simulink model "controlAerobi"  (R2017b)
settings: Solver=FixedStepDiscrete  StartTime=0.0  StopTime=inf  FixedStep=Ts  RelTol=1e-3
InitFcn:
  | load Navio2_bus;
  | Ts=0.0025;
StopFcn:
  | %save_system('controlAerobi.slx');
  | %run('D:\Eclipse_Workspaces\workspace_rasp\AutoPilot\contAerobi\UpdateFiles\CopyBuildFiles.m');
undefined symbols (not defined in the file or in its folder): DiscIntNeverNeededParam
libraries: simulink x36, sharedutil x1, sharedtransform x1, dspsigops x1
(part 3 of 4)

== system controlAerobi/Controllers/Quadrotor_Controllers/PID_cascade_controllers/PID_ATTITUDE_CONTROLLER/PID_yaw/Clamping circuit1 ==
  preSat : Inport
  postSat : Inport  Port=2
  preIntegrator : Inport  Port=3
  AND : Logic  DisableCoverage=on  OutDataTypeStr=boolean
  Abs : Abs
  Add : Sum  Inputs=+-
  Compare To Constant : simulink/Logic and Bit Operations/Compare To Constant  relop=>=  const=1e-10  OutDataTypeStr=boolean
  Equal : RelationalOperator  DisableCoverage=on  Operator===  OutDataTypeStr=boolean  RndMeth=Nearest  InputSameDT=on
  SignPreIntegrator : Signum  DisableCoverage=on
  SignPreSat : Signum  DisableCoverage=on
  Clamp : Outport
  wires:
  Abs/1 -> Compare To Constant/1
  Add/1 -> Abs/1
  postSat/1 -> Add/2
  preSat/1 -> Add/1, SignPreSat/1
  preIntegrator/1 -> SignPreIntegrator/1
  SignPreSat/1 -> Equal/1
  Compare To Constant/1 -> AND/1
  SignPreIntegrator/1 -> Equal/2
  Equal/1 -> AND/2
  AND/1 -> Clamp/1

== system controlAerobi/Controllers/Quadrotor_Controllers/PID_cascade_controllers/PID_POSITION_CONTROLLER/XY_controller/PID_XY ==
  Error : Inport
  Reset : Inport  Port=2
  ControlParam : Inport  Port=3
  Bus Selector : BusSelector  OutputSignals=PIDgains.XYcontroller.P_pos,PIDgains.XYcontroller.I_pos,PIDgains.XYcontroller.D_pos,PIDgains.XYcontroller.Sat+_XY_pos,PIDgains.XYcontroller.Sat-_XY_pos
  Clamping circuit1 : Subsystem
  Constant : Constant  Value=0
  Constant1 : Constant  Value=0
  Discrete Derivative : simulink/Discrete/Discrete Derivative  gainval=1.0  ICPrevScaledInput=0.0  InputProcessing=Inherited  OutMin=[]  OutMax=[]  OutDataType=fixdt(1, 16)  OutScaling=2^-10  DoSatur=off
  Discrete-Time Integrator : DiscreteIntegrator  ExternalReset=rising  SampleTime=Ts  ICPrevOutput=DiscIntNeverNeededParam  ICPrevScaledInput=DiscIntNeverNeededParam
  Product : Product  RndMeth=Zero
  Product1 : Product  RndMeth=Zero
  Product2 : Product  RndMeth=Zero
  Saturation Dynamic : simulink/Discontinuities/Saturation Dynamic  OutMin=[]  OutMax=[]  OutDataTypeStr=Inherit: Same as second input  OutDataType=fixdt(1, 16)  OutScaling=2^-10  DoSatur=off
  Sum : Sum  Inputs=+++
  Switch : Switch  Criteria=u2 > Threshold
  Switch4 : Switch  Criteria=u2 ~= 0
  dxdy_des : Outport
  wires:
  Error/1 -> Switch4/1
  Switch4/1 -> Product2/2, Product/2, Product1/2
  Constant1/1 -> Switch4/3
  Bus Selector/5 -> Saturation Dynamic/3  "<Sat-_XY_pos>"
  Bus Selector/4 -> Saturation Dynamic/1  "<Sat+_XY_pos>"
  Bus Selector/3 -> Product2/1  "<D_pos>"
  Bus Selector/2 -> Product1/1  "<I_pos>"
  Bus Selector/1 -> Product/1  "<P_pos>"
  ControlParam/1 -> Bus Selector/1
  Discrete Derivative/1 -> Sum/3
  Product2/1 -> Discrete Derivative/1
  Product/1 -> Sum/1
  Sum/1 -> Saturation Dynamic/2, Clamping circuit1/1(preSat)
  Reset/1 -> Switch4/2, Discrete-Time Integrator/2
  Discrete-Time Integrator/1 -> Sum/2
  Saturation Dynamic/1 -> dxdy_des/1, Clamping circuit1/2(postSat)
  Switch/1 -> Discrete-Time Integrator/1
  Clamping circuit1/1(Clamp) -> Switch/2
  Product1/1 -> Switch/3, Clamping circuit1/3(preIntegrator)
  Constant/1 -> Switch/1

== system controlAerobi/Controllers/Quadrotor_Controllers/PID_cascade_controllers/PID_POSITION_CONTROLLER/XY_controller/PID_dXY ==
  Error : Inport
  Reset : Inport  Port=2
  ControlGains : Inport  Port=3
  Bus Selector : BusSelector  OutputSignals=PIDgains.XYcontroller.P_rate,PIDgains.XYcontroller.I_rate,PIDgains.XYcontroller.D_rate,PIDgains.XYcontroller.Sat+_rate,PIDgains.XYcontroller.Sat-_rate
  Clamping circuit1 : Subsystem
  Constant : Constant  Value=0
  Constant1 : Constant  Value=0
  Discrete Derivative : simulink/Discrete/Discrete Derivative  gainval=1.0  ICPrevScaledInput=0.0  InputProcessing=Inherited  OutMin=[]  OutMax=[]  OutDataType=fixdt(1, 16)  OutScaling=2^-10  DoSatur=off
  Discrete-Time Integrator : DiscreteIntegrator  ExternalReset=rising  SampleTime=Ts  ICPrevOutput=DiscIntNeverNeededParam  ICPrevScaledInput=DiscIntNeverNeededParam
  Product : Product  RndMeth=Zero
  Product1 : Product  RndMeth=Zero
  Product2 : Product  RndMeth=Zero
  Saturation Dynamic : simulink/Discontinuities/Saturation Dynamic  OutMin=[]  OutMax=[]  OutDataTypeStr=Inherit: Same as second input  OutDataType=fixdt(1, 16)  OutScaling=2^-10  DoSatur=off
  Sum : Sum  Inputs=+++
  Switch : Switch  Criteria=u2 > Threshold
  Switch4 : Switch  Criteria=u2 ~= 0
  Fx/Fy : Outport
  wires:
  Constant/1 -> Switch/1
  Product1/1 -> Clamping circuit1/3(preIntegrator), Switch/3
  Clamping circuit1/1(Clamp) -> Switch/2
  Switch/1 -> Discrete-Time Integrator/1
  Saturation Dynamic/1 -> Clamping circuit1/2(postSat), Fx/Fy/1
  Discrete-Time Integrator/1 -> Sum/2
  Reset/1 -> Discrete-Time Integrator/2, Switch4/2
  Sum/1 -> Clamping circuit1/1(preSat), Saturation Dynamic/2
  Product/1 -> Sum/1
  Product2/1 -> Discrete Derivative/1
  Discrete Derivative/1 -> Sum/3
  ControlGains/1 -> Bus Selector/1
  Bus Selector/1 -> Product/1  "<P_rate>"
  Bus Selector/2 -> Product1/1  "<I_rate>"
  Bus Selector/3 -> Product2/1  "<D_rate>"
  Bus Selector/4 -> Saturation Dynamic/1  "<Sat+_rate>"
  Bus Selector/5 -> Saturation Dynamic/3  "<Sat-_rate>"
  Constant1/1 -> Switch4/3
  Switch4/1 -> Product1/2, Product/2, Product2/2
  Error/1 -> Switch4/1

== system controlAerobi/Controllers/Quadrotor_Controllers/PID_cascade_controllers/PID_POSITION_CONTROLLER/XY_controller/create_references ==
  yaw : Inport
  ControlModes : Inport  Port=2
  Bus Selector1 : BusSelector  OutputSignals=RemoteControl.Pitch/Xdes,RemoteControl.Roll/Ydes,ModeControl.RESET,ModeControl.POS_HOLD,ModeControl.Pos/VelXY
  Create dXY desired : MATLAB Function  TreatAsAtomicUnit=on
  Dead Zone : DeadZone  LowerValue=-0.05  UpperValue=0.05  SaturateOnIntegerOverflow=on
  Dead Zone1 : DeadZone  LowerValue=-0.05  UpperValue=0.05  SaturateOnIntegerOverflow=on
  Gain : Gain  Gain=-3
  Gain1 : Gain  Gain=3
  Logical Operator : Logic  AllPortsSameDT=off  OutDataTypeStr=boolean
  Saturation1 : Saturate  UpperLimit=3  LowerLimit=-3
  Switch1 : Switch  Criteria=u2 ~= 0
  antiwind_up_xydes : Subsystem
  zero : Constant  Value=0
  dXY_ref : Outport
  XY_ref : Outport  Port=2
  signal : Outport  Port=3
  reset : Outport  Port=4
  <POS_HOLD> : Outport  Port=5
  <Pos/VelXY> : Outport  Port=6
  wires:
  ControlModes/1 -> Bus Selector1/1
  Gain/1 -> Create dXY desired/2(chan2)
  Gain1/1 -> Create dXY desired/3(chan3)
  Bus Selector1/3 -> Logical Operator/1  "<RESET>"
  Bus Selector1/4 -> <POS_HOLD>/1, Logical Operator/2  "<POS_HOLD>"
  Bus Selector1/1 -> Dead Zone/1  "<Pitch/Xdes>"
  Bus Selector1/2 -> Dead Zone1/1  "<Roll/Ydes>"
  Bus Selector1/5 -> Switch1/2, <Pos/VelXY>/1  "<Pos/VelXY>"
  Dead Zone/1 -> Gain/1
  Dead Zone1/1 -> Gain1/1
  Logical Operator/1 -> antiwind_up_xydes/2(reset), reset/1
  Create dXY desired/1(dXY_d) -> Saturation1/1
  Saturation1/1 -> dXY_ref/1, Switch1/1
  yaw/1 -> Create dXY desired/1(yaw)
  Switch1/1 -> antiwind_up_xydes/1(error)
  zero/1 -> Switch1/3
  antiwind_up_xydes/1(ref) -> XY_ref/1
  antiwind_up_xydes/2(signal) -> signal/1

== system controlAerobi/Controllers/Quadrotor_Controllers/PID_cascade_controllers/PID_POSITION_CONTROLLER/Z_controller/Altitude_PIDs ==
  TI : Inport
  Zdes : Inport  Port=2
  dZdes : Inport  Port=3
  ControlGains : Inport  Port=4
  DataSensor : Inport  Port=5
  ControlModes : Inport  Port=6
  Bus Creator : BusCreator  Inputs=2
  Bus Selector : BusSelector  OutputSignals=position_.Position.z,position_.Velocity.dz,attitude_.AngularPosition.roll,attitude_.AngularPosition.pitch
  Bus Selector1 : BusSelector  OutputSignals=ModeControl.ALTHOLD,ModeControl.Pos/VelZ
  Divide : Product  Inputs=*/
  PID_Z : Subsystem
  PID_dZ : Subsystem
  Product : Product  RndMeth=Zero
  Sum1 : Sum  Inputs=|+-
  Sum2 : Sum
  Sum5 : Sum  Inputs=|+-
  Switch1 : Switch  Criteria=u2 ~= 0
  Trigonometric Function : Trigonometry  Operator=cos
  Trigonometric Function1 : Trigonometry  Operator=cos
  T : Outport
  dZ_des : Outport  Port=2
  wires:
  Sum5/1 -> PID_dZ/1(Error)
  PID_Z/1(dZ_des) -> Switch1/1
  Switch1/1 -> Sum5/1, Bus Creator/2  "dZ_des"
  Bus Selector/2 -> Sum5/2  "<dz>"
  Sum1/1 -> PID_Z/1(Error)
  PID_dZ/1(Fz) -> Sum2/2
  Zdes/1 -> Sum1/1, Bus Creator/1  "Z_des"
  Bus Selector1/1 -> PID_dZ/2(Reset), PID_Z/2(Reset)  "<ALTHOLD>"
  Sum2/1 -> Divide/1
  Product/1 -> Divide/2
  Trigonometric Function/1 -> Product/1
  Trigonometric Function1/1 -> Product/2
  Divide/1 -> T/1
  TI/1 -> Sum2/1
  Bus Selector/3 -> Trigonometric Function/1  "<roll>"
  Bus Selector/4 -> Trigonometric Function1/1  "<pitch>"
  DataSensor/1 -> Bus Selector/1
  ControlGains/1 -> PID_dZ/3(ControlGains), PID_Z/3(ControlGains)
  Bus Creator/1 -> dZ_des/1
  dZdes/1 -> Switch1/3
  Bus Selector/1 -> Sum1/2  "<z>"
  ControlModes/1 -> Bus Selector1/1
  Bus Selector1/2 -> Switch1/2  "<Pos/VelZ>"

== system controlAerobi/Controllers/Quadrotor_Controllers/PID_cascade_controllers/PID_POSITION_CONTROLLER/Z_controller/calculate_altitude_des ==
  DataSensor : Inport
  ControlModes : Inport  Port=2
  Bus Selector : BusSelector  OutputSignals=PositionDesired.Zdes,ModeControl.Pos/VelZ,ModeControl.EnablePC,RemoteControl.Thrust/Zdes,ModeControl.ALTHOLD
  Bus Selector1 : BusSelector  OutputSignals=position_.Position.z
  Saturation : Saturate  UpperLimit=inf  LowerLimit=0
  Sum : Sum  Inputs=|+-
  Sum1 : Sum  Inputs=|++
  Switch : Switch  Criteria=u2 ~= 0
  altitude_fcn : MATLAB Function  TreatAsAtomicUnit=on
  and : Logic  AllPortsSameDT=off  OutDataTypeStr=boolean
  antiwind_up_dzdes : Subsystem
  antiwind_up_zdes : Subsystem
  med_thrust : Constant  Value=52.23
  T : Outport
  Zdes : Outport  Port=2
  dZdes : Outport  Port=3
  wires:
  ControlModes/1 -> Bus Selector/1
  DataSensor/1 -> Bus Selector1/1
  Bus Selector/2 -> and/1  "<Pos/VelZ>"
  Bus Selector/1 -> Switch/1  "<Zdes>"
  Bus Selector/3 -> and/2  "<EnablePC>"
  and/1 -> Switch/2
  Switch/1 -> Zdes/1
  Bus Selector/5 -> antiwind_up_zdes/2(reset), altitude_fcn/2(althold)  "<ALTHOLD>"
  Bus Selector/4 -> altitude_fcn/3(thrust), Sum/1  "<Thrust/Zdes>"
  med_thrust/1 -> Sum/2
  Bus Selector1/1 -> altitude_fcn/1(z)  "<z>"
  altitude_fcn/1(zdes) -> Sum1/2
  altitude_fcn/2(thrust_ini) -> T/1
  antiwind_up_zdes/1(I) -> Sum1/1
  Sum1/1 -> Saturation/1
  antiwind_up_dzdes/1(I) -> antiwind_up_zdes/1(error), dZdes/1
  Sum/1 -> antiwind_up_dzdes/1(error)
  Saturation/1 -> Switch/3

== system controlAerobi/Controllers/Quadrotor_Controllers/Geometric_controller/trajectory_tracking/Generate_tracking_referecnces/calculate_altitude_des/antiwind_up_dzdes ==
  error : Inport
  1-D Lookup Table : Lookup_n-D  NumberOfTableDimensions=1  BreakpointsForDimension1=[-3:0.01:3]  Table=[-3:0.01:3]  InternalRulePriority=Speed  RndMeth=Simplest  InputSameDT=on
  Dead Zone : DeadZone  LowerValue=-0.8  SaturateOnIntegerOverflow=on
  Saturation : Saturate  UpperLimit=2  LowerLimit=-2
  adapt_thrust : Gain  Gain=0.01
  dZgain : Gain  Gain=6
  I : Outport
  wires:
  error/1 -> adapt_thrust/1
  1-D Lookup Table/1 -> dZgain/1
  adapt_thrust/1 -> 1-D Lookup Table/1
  dZgain/1 -> Dead Zone/1
  Dead Zone/1 -> Saturation/1
  Saturation/1 -> I/1

== system controlAerobi/Controllers/Quadrotor_Controllers/Geometric_controller/trajectory_tracking/Generate_tracking_referecnces/calculate_altitude_des/antiwind_up_zdes ==
  error : Inport
  reset : Inport  Port=2
  Clamping circuit1 : Subsystem
  Constant : Constant  Value=0
  Discrete-Time Integrator : DiscreteIntegrator  ExternalReset=rising  InitialConditionSetting=State (most efficient)  SampleTime=Ts  ICPrevOutput=DiscIntNeverNeededParam  ICPrevScaledInput=DiscIntNeverNeededParam
  Saturation : Saturate  UpperLimit=inf  LowerLimit=-inf
  Switch1 : Switch  Criteria=u2 > Threshold
  Zgain : Gain  Gain=0.5
  I : Outport
  wires:
  Clamping circuit1/1(Clamp) -> Switch1/2
  Constant/1 -> Switch1/1
  error/1 -> Zgain/1
  Discrete-Time Integrator/1 -> Clamping circuit1/1(preSat), Saturation/1
  Switch1/1 -> Discrete-Time Integrator/1
  reset/1 -> Discrete-Time Integrator/2
  Saturation/1 -> Clamping circuit1/2(postSat), I/1
  Zgain/1 -> Clamping circuit1/3(preIntegrator), Switch1/3

== system controlAerobi/Controllers/Quadrotor_Controllers/PID_cascade_controllers/PID_POSITION_CONTROLLER/XY_controller/PID_XY/Clamping circuit1 ==
  preSat : Inport
  postSat : Inport  Port=2
  preIntegrator : Inport  Port=3
  AND : Logic  DisableCoverage=on  OutDataTypeStr=boolean
  Abs : Abs
  Add : Sum  Inputs=+-
  Compare To Constant : simulink/Logic and Bit Operations/Compare To Constant  relop=>=  const=1e-10  OutDataTypeStr=boolean
  Equal : RelationalOperator  DisableCoverage=on  Operator===  OutDataTypeStr=boolean  RndMeth=Nearest  InputSameDT=on
  SignPreIntegrator : Signum  DisableCoverage=on
  SignPreSat : Signum  DisableCoverage=on
  Clamp : Outport
  wires:
  AND/1 -> Clamp/1
  Equal/1 -> AND/2
  SignPreIntegrator/1 -> Equal/2
  Compare To Constant/1 -> AND/1
  SignPreSat/1 -> Equal/1
  preIntegrator/1 -> SignPreIntegrator/1
  preSat/1 -> SignPreSat/1, Add/1
  postSat/1 -> Add/2
  Add/1 -> Abs/1
  Abs/1 -> Compare To Constant/1

== system controlAerobi/Controllers/Quadrotor_Controllers/PID_cascade_controllers/PID_POSITION_CONTROLLER/XY_controller/PID_dXY/Clamping circuit1 ==
  preSat : Inport
  postSat : Inport  Port=2
  preIntegrator : Inport  Port=3
  AND : Logic  DisableCoverage=on  OutDataTypeStr=boolean
  Abs : Abs
  Add : Sum  Inputs=+-
  Compare To Constant : simulink/Logic and Bit Operations/Compare To Constant  relop=>=  const=1e-10  OutDataTypeStr=boolean
  Equal : RelationalOperator  DisableCoverage=on  Operator===  OutDataTypeStr=boolean  RndMeth=Nearest  InputSameDT=on
  SignPreIntegrator : Signum  DisableCoverage=on
  SignPreSat : Signum  DisableCoverage=on
  Clamp : Outport
  wires:
  Abs/1 -> Compare To Constant/1
  Add/1 -> Abs/1
  postSat/1 -> Add/2
  preSat/1 -> Add/1, SignPreSat/1
  preIntegrator/1 -> SignPreIntegrator/1
  SignPreSat/1 -> Equal/1
  Compare To Constant/1 -> AND/1
  SignPreIntegrator/1 -> Equal/2
  Equal/1 -> AND/2
  AND/1 -> Clamp/1

== system controlAerobi/Controllers/Quadrotor_Controllers/PID_cascade_controllers/PID_POSITION_CONTROLLER/XY_controller/create_references/antiwind_up_xydes ==
  error : Inport
  reset : Inport  Port=2
  Clamping circuit1 : Subsystem
  Constant : Constant  Value=0
  Discrete-Time Integrator : DiscreteIntegrator  ExternalReset=rising  InitialConditionSetting=State (most efficient)  SampleTime=Ts  ICPrevOutput=DiscIntNeverNeededParam  ICPrevScaledInput=DiscIntNeverNeededParam
  Saturation : Saturate  UpperLimit=inf  LowerLimit=-inf
  Switch1 : Switch  Criteria=u2 > Threshold
  Zgain : Gain  Gain=0.5
  antiwind_up_dzdes : Subsystem
  ref : Outport
  signal : Outport  Port=2
  wires:
  Clamping circuit1/1(Clamp) -> Switch1/2
  Constant/1 -> Switch1/1
  Discrete-Time Integrator/1 -> Clamping circuit1/1(preSat), Saturation/1
  Switch1/1 -> Discrete-Time Integrator/1
  Saturation/1 -> ref/1, Clamping circuit1/2(postSat)
  Zgain/1 -> Clamping circuit1/3(preIntegrator), Switch1/3
  error/1 -> antiwind_up_dzdes/1(error)
  antiwind_up_dzdes/1(I) -> signal/1, Zgain/1
  reset/1 -> Discrete-Time Integrator/2

== system controlAerobi/Controllers/Quadrotor_Controllers/PID_cascade_controllers/PID_POSITION_CONTROLLER/Z_controller/Altitude_PIDs/PID_Z ==
  Error : Inport
  Reset : Inport  Port=2
  ControlGains : Inport  Port=3
  Bus Selector : BusSelector  OutputSignals=PIDgains.Zcontroller.P_pos,PIDgains.Zcontroller.I_pos,PIDgains.Zcontroller.D_pos,PIDgains.Zcontroller.Sat+_pos,PIDgains.Zcontroller.Sat-_pos
  Clamping circuit1 : Subsystem
  Constant : Constant  Value=0
  Discrete Derivative : simulink/Discrete/Discrete Derivative  gainval=1.0  ICPrevScaledInput=0.0  InputProcessing=Inherited  OutMin=[]  OutMax=[]  OutDataType=fixdt(1, 16)  OutScaling=2^-10  DoSatur=off
  Discrete-Time Integrator : DiscreteIntegrator  ExternalReset=rising  SampleTime=Ts  ICPrevOutput=DiscIntNeverNeededParam  ICPrevScaledInput=DiscIntNeverNeededParam
  Product : Product  RndMeth=Zero
  Product1 : Product  RndMeth=Zero
  Product2 : Product  RndMeth=Zero
  Saturation Dynamic : simulink/Discontinuities/Saturation Dynamic  OutMin=[]  OutMax=[]  OutDataTypeStr=Inherit: Same as second input  OutDataType=fixdt(1, 16)  OutScaling=2^-10  DoSatur=off
  Sum : Sum  Inputs=+++
  Switch : Switch  Criteria=u2 > Threshold
  Switch4 : Switch  Criteria=u2 ~= 0
  dZ_des : Outport
  wires:
  Product1/1 -> Clamping circuit1/3(preIntegrator), Switch/3
  Clamping circuit1/1(Clamp) -> Switch/2
  Switch/1 -> Discrete-Time Integrator/1
  Saturation Dynamic/1 -> Clamping circuit1/2(postSat), dZ_des/1
  Discrete-Time Integrator/1 -> Sum/2
  Reset/1 -> Switch4/2, Discrete-Time Integrator/2
  Sum/1 -> Clamping circuit1/1(preSat), Saturation Dynamic/2
  Product/1 -> Sum/1
  Product2/1 -> Discrete Derivative/1
  Discrete Derivative/1 -> Sum/3
  ControlGains/1 -> Bus Selector/1
  Bus Selector/1 -> Product/1  "<P_pos>"
  Bus Selector/2 -> Product1/1  "<I_pos>"
  Bus Selector/3 -> Product2/1  "<D_pos>"
  Bus Selector/4 -> Saturation Dynamic/1  "<Sat+_pos>"
  Bus Selector/5 -> Saturation Dynamic/3  "<Sat-_pos>"
  Constant/1 -> Switch4/3, Switch/1
  Switch4/1 -> Product1/2, Product/2, Product2/2
  Error/1 -> Switch4/1

== system controlAerobi/Controllers/Quadrotor_Controllers/PID_cascade_controllers/PID_POSITION_CONTROLLER/Z_controller/Altitude_PIDs/PID_dZ ==
  Error : Inport
  Reset : Inport  Port=2
  ControlGains : Inport  Port=3
  Bus Selector : BusSelector  OutputSignals=PIDgains.Zcontroller.P_rate,PIDgains.Zcontroller.I_rate,PIDgains.Zcontroller.D_rate,PIDgains.Zcontroller.Sat+_rate,PIDgains.Zcontroller.Sat-_rate
  Clamping circuit1 : Subsystem
  Constant : Constant  Value=0
  Discrete Derivative : simulink/Discrete/Discrete Derivative  gainval=1.0  ICPrevScaledInput=0.0  InputProcessing=Inherited  OutMin=[]  OutMax=[]  OutDataType=fixdt(1, 16)  OutScaling=2^-10  DoSatur=off
  Discrete-Time Integrator : DiscreteIntegrator  ExternalReset=rising  SampleTime=Ts  ICPrevOutput=DiscIntNeverNeededParam  ICPrevScaledInput=DiscIntNeverNeededParam
  Product : Product  RndMeth=Zero
  Product1 : Product  RndMeth=Zero
  Product2 : Product  RndMeth=Zero
  Saturation Dynamic : simulink/Discontinuities/Saturation Dynamic  OutMin=[]  OutMax=[]  OutDataTypeStr=Inherit: Same as second input  OutDataType=fixdt(1, 16)  OutScaling=2^-10  DoSatur=off
  Sum : Sum  Inputs=+++
  Switch : Switch  Criteria=u2 > Threshold
  Switch4 : Switch  Criteria=u2 ~= 0
  Fz : Outport
  wires:
  Error/1 -> Switch4/1
  Switch4/1 -> Product2/2, Product/2, Product1/2
  Constant/1 -> Switch4/3, Switch/1
  Bus Selector/5 -> Saturation Dynamic/3  "<Sat-_rate>"
  Bus Selector/4 -> Saturation Dynamic/1  "<Sat+_rate>"
  Bus Selector/3 -> Product2/1  "<D_rate>"
  Bus Selector/2 -> Product1/1  "<I_rate>"
  Bus Selector/1 -> Product/1  "<P_rate>"
  ControlGains/1 -> Bus Selector/1
  Discrete Derivative/1 -> Sum/3
  Product2/1 -> Discrete Derivative/1
  Product/1 -> Sum/1
  Sum/1 -> Saturation Dynamic/2, Clamping circuit1/1(preSat)
  Reset/1 -> Discrete-Time Integrator/2, Switch4/2
  Discrete-Time Integrator/1 -> Sum/2
  Saturation Dynamic/1 -> Fz/1, Clamping circuit1/2(postSat)
  Switch/1 -> Discrete-Time Integrator/1
  Clamping circuit1/1(Clamp) -> Switch/2
  Product1/1 -> Switch/3, Clamping circuit1/3(preIntegrator)

== system controlAerobi/Controllers/Quadrotor_Controllers/PID_cascade_controllers/PID_POSITION_CONTROLLER/Z_controller/calculate_altitude_des/antiwind_up_dzdes ==
  error : Inport
  1-D Lookup Table : Lookup_n-D  NumberOfTableDimensions=1  BreakpointsForDimension1=[-3:0.01:3]  Table=[-3:0.01:3]  InternalRulePriority=Speed  RndMeth=Simplest  InputSameDT=on
  Dead Zone : DeadZone  LowerValue=-0.8  SaturateOnIntegerOverflow=on
  Saturation : Saturate  UpperLimit=2  LowerLimit=-2
  adapt_thrust : Gain  Gain=0.01
  dZgain : Gain  Gain=6
  I : Outport
  wires:
  error/1 -> adapt_thrust/1
  1-D Lookup Table/1 -> dZgain/1
  adapt_thrust/1 -> 1-D Lookup Table/1
  dZgain/1 -> Dead Zone/1
  Dead Zone/1 -> Saturation/1
  Saturation/1 -> I/1

== system controlAerobi/Controllers/Quadrotor_Controllers/PID_cascade_controllers/PID_POSITION_CONTROLLER/Z_controller/calculate_altitude_des/antiwind_up_zdes ==
  error : Inport
  reset : Inport  Port=2
  Clamping circuit1 : Subsystem
  Constant : Constant  Value=0
  Discrete-Time Integrator : DiscreteIntegrator  ExternalReset=rising  InitialConditionSetting=State (most efficient)  SampleTime=Ts  ICPrevOutput=DiscIntNeverNeededParam  ICPrevScaledInput=DiscIntNeverNeededParam
  Saturation : Saturate  UpperLimit=inf  LowerLimit=-inf
  Switch1 : Switch  Criteria=u2 > Threshold
  Zgain : Gain  Gain=0.5
  I : Outport
  wires:
  Clamping circuit1/1(Clamp) -> Switch1/2
  Constant/1 -> Switch1/1
  error/1 -> Zgain/1
  Discrete-Time Integrator/1 -> Clamping circuit1/1(preSat), Saturation/1
  Switch1/1 -> Discrete-Time Integrator/1
  reset/1 -> Discrete-Time Integrator/2
  Saturation/1 -> Clamping circuit1/2(postSat), I/1
  Zgain/1 -> Clamping circuit1/3(preIntegrator), Switch1/3

== system controlAerobi/Controllers/Quadrotor_Controllers/Geometric_controller/trajectory_tracking/Generate_tracking_referecnces/calculate_altitude_des/antiwind_up_zdes/Clamping circuit1 ==
  preSat : Inport
  postSat : Inport  Port=2
  preIntegrator : Inport  Port=3
  AND : Logic  DisableCoverage=on  OutDataTypeStr=boolean
  Abs : Abs
  Add : Sum  Inputs=+-
  Compare To Constant : simulink/Logic and Bit Operations/Compare To Constant  relop=>=  const=1e-10  OutDataTypeStr=boolean
  Equal : RelationalOperator  DisableCoverage=on  Operator===  OutDataTypeStr=boolean  RndMeth=Nearest  InputSameDT=on
  SignPreIntegrator : Signum  DisableCoverage=on
  SignPreSat : Signum  DisableCoverage=on
  Clamp : Outport
  wires:
  Abs/1 -> Compare To Constant/1
  Add/1 -> Abs/1
  postSat/1 -> Add/2
  preSat/1 -> Add/1, SignPreSat/1
  preIntegrator/1 -> SignPreIntegrator/1
  SignPreSat/1 -> Equal/1
  Compare To Constant/1 -> AND/1
  SignPreIntegrator/1 -> Equal/2
  Equal/1 -> AND/2
  AND/1 -> Clamp/1

== system controlAerobi/Controllers/Quadrotor_Controllers/PID_cascade_controllers/PID_POSITION_CONTROLLER/XY_controller/create_references/antiwind_up_xydes/Clamping circuit1 ==
  preSat : Inport
  postSat : Inport  Port=2
  preIntegrator : Inport  Port=3
  AND : Logic  DisableCoverage=on  OutDataTypeStr=boolean
  Abs : Abs
  Add : Sum  Inputs=+-
  Compare To Constant : simulink/Logic and Bit Operations/Compare To Constant  relop=>=  const=1e-10  OutDataTypeStr=boolean
  Equal : RelationalOperator  DisableCoverage=on  Operator===  OutDataTypeStr=boolean  RndMeth=Nearest  InputSameDT=on
  SignPreIntegrator : Signum  DisableCoverage=on
  SignPreSat : Signum  DisableCoverage=on
  Clamp : Outport
  wires:
  Abs/1 -> Compare To Constant/1
  Add/1 -> Abs/1
  postSat/1 -> Add/2
  preSat/1 -> Add/1, SignPreSat/1
  preIntegrator/1 -> SignPreIntegrator/1
  SignPreSat/1 -> Equal/1
  Compare To Constant/1 -> AND/1
  SignPreIntegrator/1 -> Equal/2
  Equal/1 -> AND/2
  AND/1 -> Clamp/1

== system controlAerobi/Controllers/Quadrotor_Controllers/PID_cascade_controllers/PID_POSITION_CONTROLLER/XY_controller/create_references/antiwind_up_xydes/antiwind_up_dzdes ==
  error : Inport
  1-D Lookup Table : Lookup_n-D  NumberOfTableDimensions=1  BreakpointsForDimension1=[-3:0.01:3]  Table=[-3:0.01:3]  InternalRulePriority=Speed  RndMeth=Simplest  InputSameDT=on
  Dead Zone : DeadZone  LowerValue=-0.2  UpperValue=0.2  SaturateOnIntegerOverflow=on
  Saturation : Saturate  UpperLimit=inf  LowerLimit=-inf
  adapt_thrust : Gain
  dZgain : Gain  Gain=10
  I : Outport
  wires:
  error/1 -> adapt_thrust/1
  1-D Lookup Table/1 -> dZgain/1
  adapt_thrust/1 -> 1-D Lookup Table/1
  dZgain/1 -> Dead Zone/1
  Dead Zone/1 -> Saturation/1
  Saturation/1 -> I/1

== system controlAerobi/Controllers/Quadrotor_Controllers/PID_cascade_controllers/PID_POSITION_CONTROLLER/Z_controller/Altitude_PIDs/PID_Z/Clamping circuit1 ==
  preSat : Inport
  postSat : Inport  Port=2
  preIntegrator : Inport  Port=3
  AND : Logic  DisableCoverage=on  OutDataTypeStr=boolean
  Abs : Abs
  Add : Sum  Inputs=+-
  Compare To Constant : simulink/Logic and Bit Operations/Compare To Constant  relop=>=  const=1e-10  OutDataTypeStr=boolean
  Equal : RelationalOperator  DisableCoverage=on  Operator===  OutDataTypeStr=boolean  RndMeth=Nearest  InputSameDT=on
  SignPreIntegrator : Signum  DisableCoverage=on
  SignPreSat : Signum  DisableCoverage=on
  Clamp : Outport
  wires:
  Abs/1 -> Compare To Constant/1
  Add/1 -> Abs/1
  postSat/1 -> Add/2
  preSat/1 -> Add/1, SignPreSat/1
  preIntegrator/1 -> SignPreIntegrator/1
  SignPreSat/1 -> Equal/1
  Compare To Constant/1 -> AND/1
  SignPreIntegrator/1 -> Equal/2
  Equal/1 -> AND/2
  AND/1 -> Clamp/1

== system controlAerobi/Controllers/Quadrotor_Controllers/PID_cascade_controllers/PID_POSITION_CONTROLLER/Z_controller/Altitude_PIDs/PID_dZ/Clamping circuit1 ==
  preSat : Inport
  postSat : Inport  Port=2
  preIntegrator : Inport  Port=3
  AND : Logic  DisableCoverage=on  OutDataTypeStr=boolean
  Abs : Abs
  Add : Sum  Inputs=+-
  Compare To Constant : simulink/Logic and Bit Operations/Compare To Constant  relop=>=  const=1e-10  OutDataTypeStr=boolean
  Equal : RelationalOperator  DisableCoverage=on  Operator===  OutDataTypeStr=boolean  RndMeth=Nearest  InputSameDT=on
  SignPreIntegrator : Signum  DisableCoverage=on
  SignPreSat : Signum  DisableCoverage=on
  Clamp : Outport
  wires:
  AND/1 -> Clamp/1
  Equal/1 -> AND/2
  SignPreIntegrator/1 -> Equal/2
  Compare To Constant/1 -> AND/1
  SignPreSat/1 -> Equal/1
  preIntegrator/1 -> SignPreIntegrator/1
  preSat/1 -> SignPreSat/1, Add/1
  postSat/1 -> Add/2
  Add/1 -> Abs/1
  Abs/1 -> Compare To Constant/1

== system controlAerobi/Controllers/Quadrotor_Controllers/PID_cascade_controllers/PID_POSITION_CONTROLLER/Z_controller/calculate_altitude_des/antiwind_up_zdes/Clamping circuit1 ==
  preSat : Inport
  postSat : Inport  Port=2
  preIntegrator : Inport  Port=3
  AND : Logic  DisableCoverage=on  OutDataTypeStr=boolean
  Abs : Abs
  Add : Sum  Inputs=+-
  Compare To Constant : simulink/Logic and Bit Operations/Compare To Constant  relop=>=  const=1e-10  OutDataTypeStr=boolean
  Equal : RelationalOperator  DisableCoverage=on  Operator===  OutDataTypeStr=boolean  RndMeth=Nearest  InputSameDT=on
  SignPreIntegrator : Signum  DisableCoverage=on
  SignPreSat : Signum  DisableCoverage=on
  Clamp : Outport
  wires:
  Abs/1 -> Compare To Constant/1
  Add/1 -> Abs/1
  postSat/1 -> Add/2
  preSat/1 -> Add/1, SignPreSat/1
  preIntegrator/1 -> SignPreIntegrator/1
  SignPreSat/1 -> Equal/1
  Compare To Constant/1 -> AND/1
  SignPreIntegrator/1 -> Equal/2
  Equal/1 -> AND/2
  AND/1 -> Clamp/1

== matlab function controlAerobi/Controllers/Quadrotor_Controllers/PID_cascade_controllers/PID_POSITION_CONTROLLER/Z_controller/calculate_altitude_des/altitude_fcn ==
  data: z input; zdes output; althold input; thrust input; thrust_ini output
function [zdes,thrust_ini] = altitude_fcn(z,althold,thrust)

persistent z0 althold0 thrust0
if isempty(z0)||isempty(althold0)||isempty(thrust0)
    z0 = z;
    althold0 = 0;
    thrust0 = thrust;

else
    if althold0 == 0 && althold == 1
        z0 = z; 
        thrust0 = thrust;  
    end
    althold0 = double(althold);      
end

zdes = z0;
thrust_ini = thrust0;

== matlab function controlAerobi/Controllers/Quadrotor_Controllers/PID_cascade_controllers/PID_ATTITUDE_CONTROLLER/Continuous Yaw Generator ==
  data: yaw_position input; yaw_desired output; yaw output; reset input; increment input
function [yaw_desired,yaw] = ContinuousYawGenerator(yaw_position, reset, increment)
%%This function convert the discontinuous 
%%yaw signal [-PI,PI] into a continuous signal [-inf,inf].
persistent yaw_references yaw_position_old n
if isempty(yaw_references)||isempty(yaw_position_old)||isempty(n)
    yaw_references=0;
    yaw_position_old=yaw_position;
    n=0; %number of spins
else
    if reset==0
        yaw_references=yaw_position+n*2*pi; %while the controller is inactive the position desired is equal to the actual position.
    else
        %count the number of spins 
        if yaw_position-yaw_position_old<-pi 
            n = n+1;
        elseif yaw_position-yaw_position_old>pi
            n = n-1;
        end    
        yaw_position_old=yaw_position;
        yaw_references=yaw_references+increment*(1.5/100);
    end
end
yaw=yaw_position+n*2*pi; % this line changes the negative gains values of the yaw control position
yaw_desired = yaw_references;

== matlab function controlAerobi/Controllers/Quadrotor_Controllers/Geometric_controller/attitude_tracking/attitude_geometric_control ==
  data: roll input; U2 output; pitch input; yaw input; droll input; dpitch input; dyaw input; R_d input; Omega_d input; dOmega_d input; reset input; J input; k_R input; k_Omega input; k_I input; c2 input; sat input; U3 output; U4 output; drift input
function [U2,U3,U4] = attitude_geometric_control(roll,pitch,yaw,droll,dpitch,dyaw,R_d,Omega_d,dOmega_d,reset,J,k_R,k_Omega,k_I,c2,sat,drift) 

%-J inertia matrix
%-R rotation matrix
%-Omega angular velocity
persistent e_I M
if isempty(e_I)||isempty(M)
    e_I = [0;0;0];
    M = [0;0;0];
end
dt = 0.0025;
R = [ cos(pitch)*cos(yaw)  -cos(roll)*sin(yaw)+sin(roll)*sin(pitch)*cos(yaw)   sin(roll)*sin(yaw)+cos(roll)*sin(pitch)*cos(yaw);
      cos(pitch)*sin(yaw)  cos(roll)*cos(yaw)+sin(roll)*sin(pitch)*sin(yaw)   -sin(roll)*cos(yaw)+cos(roll)*sin(pitch)*sin(yaw);
               -sin(pitch)                             sin(roll)*cos(pitch)                               cos(roll)*cos(pitch)];

%The attitude tracking error e_R is given by:
Re_R = 0.5*(R_d'*R-R'*R_d);
e_R = [Re_R(3,2);Re_R(1,3);Re_R(2,1)];

%The tracking error for the angular velocity is defined as:
Omega = [droll;dpitch;dyaw];
e_Omega = Omega - R'*R_d*Omega_d;

%The integral error e_I is given by:
if reset == 1
    e_I = 0.5*(e_Omega + diag(c2)*e_R)*dt - e_I;
    for i=1:3
        if M(i) > sat(i) || M(i) < -sat(i)
            k_I(i) = 0;
        end
    end
else
    e_I = [0;0;0];
end

%Then the control inputs are chosen as follows:
% Omega_sk = [       0 -Omega(3) Omega(2);
%              Omega(3)       0 -Omega(1);
%             -Omega(2) Omega(1)       0];

RtRdOmegad =  R'*R_d*Omega_d;
RtRdOmegad_sk = [           0   -RtRdOmegad(3)    RtRdOmegad(2);
                 RtRdOmegad(3)              0    -RtRdOmegad(1);
                -RtRdOmegad(2)   RtRdOmegad(1)               0];

%M = -diag(k_R)*e_R -diag(k_Omega)*e_Omega + cross(Omega,J*Omega) - J*(Omega_sk*R'*R_d*Omega_d - R'*R_d*dOmega_d) + drift;
M = -diag(k_R)*e_R -diag(k_Omega)*e_Omega -diag(k_I)*e_I + RtRdOmegad_sk*J*R'*R_d*Omega_d + J*R'*R_d*dOmega_d + drift;


U2 = M(1);
U3 = M(2);
U4 = M(3);
end

== matlab function controlAerobi/Controllers/Quadrotor_Controllers/Geometric_controller/attitude_tracking/Generate_attitude_refereces/Calculate_rotation_matrix_des ==
  data: roll input; R_d output; pitch input; yaw input
function R_d = rotationMatrix(roll,pitch,yaw)

R_d =  [ cos(pitch)*cos(yaw)  -cos(roll)*sin(yaw)+sin(roll)*sin(pitch)*cos(yaw)   sin(roll)*sin(yaw)+cos(roll)*sin(pitch)*cos(yaw);
         cos(pitch)*sin(yaw)  cos(roll)*cos(yaw)+sin(roll)*sin(pitch)*sin(yaw)   -sin(roll)*cos(yaw)+cos(roll)*sin(pitch)*sin(yaw);
                 -sin(pitch)                              sin(roll)*cos(pitch)                               cos(roll)*cos(pitch)];
           
end

== matlab function controlAerobi/Controllers/Quadrotor_Controllers/Geometric_controller/trajectory_tracking/Generate_tracking_referecnces/Calculate_position_des/Create dXY desired ==
  data: yaw input; chan2 input; chan3 input; dXY_d output
function dXY_d = dXYdesired(yaw,chan2,chan3)

R = [cos(yaw) -sin(yaw);sin(yaw) cos(yaw)];

dXY_d = R*[chan2;chan3];

== matlab function controlAerobi/Controllers/Quadrotor_Controllers/Geometric_controller/attitude_tracking/Generate_attitude_refereces/MATLAB Function ==
  data: roll input; Omega_d output; pitch input; yaw input
function Omega_d = cal_omega_des(roll,pitch,yaw)

KQ = [0 0.000025 0 0.000025 0 0.000025];
KR = [10; 10; 10];
T = 0.0025;
persistent  x_k P_k
if isempty(x_k) || isempty(P_k)
    x_k = [0;0;0;0;0;0];  
    P_k = eye(6,6);

else
    F = [1 T 0 0 0 0;
         0 1 0 0 0 0;
         0 0 1 T 0 0;
         0 0 0 1 0 0;
         0 0 0 0 1 T;
         0 0 0 0 0 1];

    z_k = [roll;pitch;yaw];
    y_k = [x_k(1);x_k(3);x_k(5)];
    H =[1   0  0  0  0  0;
        0   0  1  0  0  0;
        0   0  0  0  1  0];
    
    %B = [1 0 0; 0 1 0];
    Q = diag(KQ);
    R = diag(KR);
%---------PREDICTION---------%
%1. Project the state ahead
    x_k = F * x_k;% + B * Acc_z;
%2. Project the error covariance ahead
    P_k = F * P_k * F' + Q;  
%--------CORRECTION----------%
%1. Compute the Kalman Gain
    K_k = P_k * H' / (H*P_k*H' + R);
    %resid = [sqrt(x0^2+y0^2);atan2(y0,x0);z0] - y_k;
    resid = z_k - y_k;
%2. Update the estimate via measurement
    x_k = x_k + K_k * resid;
%3. Update the error covariance
    P_k = (eye(size(K_k,1)) - K_k * H) * P_k;
end

droll = x_k(2);
dpitch = x_k(4);
dyaw = x_k(6);

Omega_d = [-sin(pitch)*dyaw+droll;
            cos(pitch)*sin(roll)*dyaw+cos(roll)*dpitch;
            -sin(roll)*dpitch+cos(pitch)*cos(roll)*dyaw];

== matlab function controlAerobi/Controllers/Quadrotor_Controllers/Geometric_controller/trajectory_tracking/trajectory_tracking ==
  data: roll input; f output; pitch input; yaw input; px input; py input; pz input; vx input; vy input; vz input; x_d input; v_d input; ddx_d input; b1_d input; T input; reset input; k_x input; k_v input; k_i input; c1 input; sat input; m input; R_d output
function [f,R_d] = trajectory_tracking_control(roll,pitch,yaw,px,py,pz,vx,vy,vz,x_d,v_d,ddx_d,b1_d,T,reset,k_x,k_v,k_i,c1,sat,m)

g = -9.81;
R = [ cos(pitch)*cos(yaw)  -cos(roll)*sin(yaw)+sin(roll)*sin(pitch)*cos(yaw)   sin(roll)*sin(yaw)+cos(roll)*sin(pitch)*cos(yaw);
      cos(pitch)*sin(yaw)  cos(roll)*cos(yaw)+sin(roll)*sin(pitch)*sin(yaw)   -sin(roll)*cos(yaw)+cos(roll)*sin(pitch)*sin(yaw);
               -sin(pitch)                             sin(roll)*cos(pitch)                               cos(roll)*cos(pitch)];
dt = 0.0025;
persistent e_i M
if isempty(e_i)||isempty(M)
    e_i = [0;0;0];
    M = [0;0;0];
end
           
x = [px;py;pz];
e_x = x - x_d;

v = [vx;vy;vz];
e_v = v - v_d;

%The integral error e_I is given by:
if reset == 1
    e_i = 0.5*(e_v + diag(c1)*e_x)*dt - e_i;
    for i=1:3
        if M(i) > sat(i) || M(i) < -sat(i)
            k_i(i) = 0;
        end
    end
else
    e_i = [0;0;0];
end

e3 = [0;0;1];

control =  -diag(k_x)*e_x-diag(k_v)*e_v-diag(k_i)*e_i-m*g*e3+m*ddx_d;
b3_d = (control)/norm(control);
b2_d = cross(b3_d,b1_d)/norm(cross(b3_d,b1_d));
R_d = [cross(b2_d,b3_d),b2_d,b3_d];
f = control'/(R*e3)'+T/(cos(roll)*cos(pitch));

== matlab function controlAerobi/Controllers/Quadrotor_Controllers/PID_cascade_controllers/PID_POSITION_CONTROLLER/XY_controller/Create_Pos_Hold ==
  data: solution input; XY input; XY_ref input; signal input; XYd output; enable input
function XYd = createPosHold(solution,XY,XY_ref,signal,enable)

persistent posHold posState stop XY_ref0 solution0
if isempty(posHold)||isempty(posState)||isempty(stop)||isempty(XY_ref0)||isempty(solution0)
    posHold=XY;
    posState = 0;
    stop = [0;0];
    XY_ref0 = [0;0];
    solution0 = solution;
else
    if enable == 0 && posState == 0 %New
        posHold = XY; 
        XY_ref0 = [0;0];
    elseif posState == 0 && enable == 1 
        posHold = XY;
        XY_ref0 = [0;0];
    elseif posState == 1
        if solution0 ~= solution
            posHold = XY;
            XY_ref0 = XY_ref;
        end
        for i=1:2
            if signal(i) == 0 && stop(i) == 0
                posHold(i) = XY(i); 
                stop(i) = 1;
                XY_ref0(i) = XY_ref(i);
            elseif abs(signal(i)) > 0 && stop(i) == 1
                stop(i) = 0;
            end
        end
    end
    posState = double(enable);
            
end  

if enable == 0
    XYd = posHold;
else
    XYd = posHold + XY_ref-XY_ref0;
end

== matlab function controlAerobi/Controllers/Quadrotor_Controllers/Geometric_controller/attitude_tracking/Generate_attitude_refereces/calculate_dOmega_d ==
  data: Omegad input; dOmega_d output
function dOmega_d = dOmegadesired(Omegad)

KQ = [0 0.0025 0 0.0025 0 0.0025];
KR = [0.01; 0.01; 0.01];
T = 0.0025;
persistent  x_k P_k
if isempty(x_k) || isempty(P_k)
    x_k = [0;0;0;0;0;0];  
    P_k = eye(6,6);

else
    F = [1 T 0 0 0 0;
         0 1 0 0 0 0;
         0 0 1 T 0 0;
         0 0 0 1 0 0;
         0 0 0 0 1 T;
         0 0 0 0 0 1];

    z_k = Omegad;
    y_k = [x_k(1);x_k(3);x_k(5)];
    H =[1   0  0  0  0  0;
        0   0  1  0  0  0;
        0   0  0  0  1  0];
    
    %B = [1 0 0; 0 1 0];
    Q = diag(KQ);
    R = diag(KR);
%---------PREDICTION---------%
%1. Project the state ahead
    x_k = F * x_k;% + B * Acc_z;
%2. Project the error covariance ahead
    P_k = F * P_k * F' + Q;  
%--------CORRECTION----------%
%1. Compute the Kalman Gain
    K_k = P_k * H' / (H*P_k*H' + R);
    %resid = [sqrt(x0^2+y0^2);atan2(y0,x0);z0] - y_k;
    resid = z_k - y_k;
%2. Update the estimate via measurement
    x_k = x_k + K_k * resid;
%3. Update the error covariance
    P_k = (eye(size(K_k,1)) - K_k * H) * P_k;
end

dOmega_d =[x_k(2);x_k(4);x_k(6)];

== matlab function controlAerobi/Controllers/Quadrotor_Controllers/Geometric_controller/trajectory_tracking/Generate_tracking_referecnces/calculate_v_d ==
  data: x_d input; v_d output
function v_d = cal_x_des(x_d)

KQ = [0 0.000025 0 0.000025 0 0.000025];
KR = [10; 10; 10];
T = 0.0025;
persistent  x_k P_k
if isempty(x_k) || isempty(P_k)
    x_k = [0;0;0;0;0;0];  
    P_k = eye(6,6);

else
    F = [1 T 0 0 0 0;
         0 1 0 0 0 0;
         0 0 1 T 0 0;
         0 0 0 1 0 0;
         0 0 0 0 1 T;
         0 0 0 0 0 1];

    z_k = [x_d(1);x_d(2);x_d(3)];
    y_k = [x_k(1);x_k(3);x_k(5)];
    H =[1   0  0  0  0  0;
        0   0  1  0  0  0;
        0   0  0  0  1  0];
    
    %B = [1 0 0; 0 1 0];
    Q = diag(KQ);
    R = diag(KR);
%---------PREDICTION---------%
%1. Project the state ahead
    x_k = F * x_k;% + B * Acc_z;
%2. Project the error covariance ahead
    P_k = F * P_k * F' + Q;  
%--------CORRECTION----------%
%1. Compute the Kalman Gain
    K_k = P_k * H' / (H*P_k*H' + R);
    %resid = [sqrt(x0^2+y0^2);atan2(y0,x0);z0] - y_k;
    resid = z_k - y_k;
%2. Update the estimate via measurement
    x_k = x_k + K_k * resid;
%3. Update the error covariance
    P_k = (eye(size(K_k,1)) - K_k * H) * P_k;
end

v_d = [x_k(2);x_k(4);x_k(6)];

== matlab function controlAerobi/Sensors/position/EKF_total_Station_Lidar/filter/buffer ==
  data: x_ output; x input; y input; z input; y_ output; z_ output; acc_hat output; freq output; a_b input
function [x_,y_,z_,acc_hat,freq] = data_buffer(x,y,z,a_b)

dt = 0.0025;
persistent buffer time index counter acc_
if isempty(buffer)||isempty(time)||isempty(index)||isempty(counter)||isempty(acc_)
    buffer = zeros(3,20);
    time = 0;
    index = 1;
    counter = zeros(1,20);
    buffer(:,index) = [x;y;z];
    counter(1) = 1;   
    acc_ = [0;0;1];
else
    alpha = 0.2;
    a_b = a_b/norm(a_b);
    acc_ = (a_b * alpha) + (acc_ * (1.0 - alpha));
    time = time + dt;
    if time > 0.05
        time = 0;
        if (buffer(1,index) ~= x || buffer(2,index) ~= y )
            buffer(:,index) = [x;y;z];
            counter(index) = 1;
        else

            buffer(:,index) = [x;y;z];
            counter(index) = 0;
        end
        if index == 20
            index = 1;
        else
            index = index + 1;
        end

    end
    
end
    freq =sum(counter);
    if freq > 20
        freq = 20;
    end
    if isnan(x) || isnan(y) || isinf(x) || isinf(y) || abs(x) > 50 || abs(y) > 50
        if index <= 1
            x_ = buffer(1,20);
            y_ = buffer(2,20);
        else       
            x_ = buffer(1,index-1);
            y_ = buffer(2,index-1);
        end
        z_ = z;
    else
        if z < 0.35
            z_ = 0.35;
        else
            z_ = z;
        end
        x_ = x;
        y_ = y;   
    end
    acc_hat = acc_;
end

== matlab function controlAerobi/Controllers/Quadrotor_Controllers/Geometric_controller/trajectory_tracking/Generate_tracking_referecnces/calculate_altitude_des/altitude_fcn ==
  data: z input; zdes output; althold input; thrust input; thrust_ini output
function [zdes,thrust_ini] = altitude_fcn(z,althold,thrust)

persistent z0 althold0 thrust0
if isempty(z0)||isempty(althold0)||isempty(thrust0)
    z0 = z;
    althold0 = 0;
    thrust0 = thrust;

else
    if althold0 == 0 && althold == 1
        z0 = z; 
        thrust0 = thrust;
    elseif althold0 == 0 && althold == 0
        z0 = z;
    end
    althold0 = double(althold);      
end

zdes = z0;
thrust_ini = thrust0;

== matlab function controlAerobi/Controllers/Quadrotor_Controllers/Geometric_controller/trajectory_tracking/Generate_tracking_referecnces/calculate_ddx_d ==
  data: v_d input; ddx_d output
function ddx_d = calc_ddx_des(v_d)

KQ = [0 0.0025 0 0.0025 0 0.0025];
KR = [1; 1; 1];
T = 0.0025;
persistent  x_k P_k
if isempty(x_k) || isempty(P_k)
    x_k = [0;0;0;0;0;0];  
    P_k = eye(6,6);

else
    F = [1 T 0 0 0 0;
         0 1 0 0 0 0;
         0 0 1 T 0 0;
         0 0 0 1 0 0;
         0 0 0 0 1 T;
         0 0 0 0 0 1];

    z_k = v_d;
    y_k = [x_k(1);x_k(3);x_k(5)];
    H =[1   0  0  0  0  0;
        0   0  1  0  0  0;
        0   0  0  0  1  0];
    
    %B = [1 0 0; 0 1 0];
    Q = diag(KQ);
    R = diag(KR);
%---------PREDICTION---------%
%1. Project the state ahead
    x_k = F * x_k;% + B * Acc_z;
%2. Project the error covariance ahead
    P_k = F * P_k * F' + Q;  
%--------CORRECTION----------%
%1. Compute the Kalman Gain
    K_k = P_k * H' / (H*P_k*H' + R);
    %resid = [sqrt(x0^2+y0^2);atan2(y0,x0);z0] - y_k;
    resid = z_k - y_k;
%2. Update the estimate via measurement
    x_k = x_k + K_k * resid;
%3. Update the error covariance
    P_k = (eye(size(K_k,1)) - K_k * H) * P_k;
end

ddx_d =[x_k(2);x_k(4);x_k(6)];

== matlab function controlAerobi/Sensors/position/EKF_total_Station_Lidar/filter/Liner Fixed-gain Filter ==
  data: thrust input; dx input; dy input; freq input; roll input; pitch input; yaw input; a_b input; vx output; vy output
function [vx,vy] = linear_Fixed_Gain_Filter(thrust,dx,dy,freq,roll,pitch,yaw,a_b)

dt = 0.0025;
m = 2.5;
mu = 0.87;
R_yaw = [cos(yaw) -sin(yaw);sin(yaw) cos(yaw)];  
persistent x_k P_k
if isempty(x_k)||isempty(P_k)
    x_k = [0;0];
    P_k = [1 0;0 1;];
        
else
    if thrust < 40
        thrust = 40;
    elseif thrust >120
        thrust = 120;
    end
    u = 62.5/thrust;
    
    
    a_I = [a_b(2)-sin(pitch);
           -a_b(1)-sin(roll)*cos(pitch);
           a_b(3)-cos(roll)*cos(pitch)];

      
    x_I = R_yaw*[dx;dy];
    
    F = [(mu*u)/m          0;
                0   (mu*u)/m];
    
    H = [(mu*u)/m          0; 
                0   (mu*u)/m; 
                dt          0;
                0          dt;];
            
    Q = diag([1 1]);
    if freq >= 20
        R = diag([0.5 0.5 0.004 0.004]);
    else
        R = diag([0.01 0.01 100000 100000]);
    end
    
    z_k = [a_I(1);a_I(2);x_I(1);x_I(2)];
    y_k = x_k;
        %---------PREDICTION---------%
    %1. Project the state ahead
        x_k = F * x_k;% + B * w_k;
    %2. Project the error covariance ahead
        P_k = F * P_k * F' + Q;  
    %--------CORRECTION----------%
    %1. Compute the Kalman Gain
        K_k = P_k * H' / (H*P_k*H' + R);
        
        resid = z_k - H*y_k;
    %2. Update the estimate via measurement
        x_k = x_k + K_k * resid;
    %3. Update the error covariance
        P_k = (eye(size(K_k,1)) - K_k * H) * P_k;    
    
 
end
v = R_yaw'*x_k;
vx = v(1);
vy = v(2);

== matlab function controlAerobi/Sensors/attitude/AttitudeEstimator/calib gyro lsm/MATLAB Function ==
  data: g input; g_offset output
function g_offset = gyro_offset(g)

persistent offset num suma
if isempty(offset)||isempty(num)||isempty(suma)
    suma = [0;0;0];
    offset = [0;0;0];
    num = 0;
else
    if abs(norm(g))<0.2
        suma = suma+g;
        num = num+1;
    else
        suma = [0;0;0];
        num = 0;
    end

    if num == 200
        offset = suma/num;
        num = 0;
        suma = [0;0;0];
    end
end
g_offset =g - offset;

== matlab function controlAerobi/Sensors/position/EKF_total_Station_Lidar/filter/EKF_dXYZ ==
  data: timeTS input; x input; y input; z input; a_b input; roll input; pitch input; yaw input; dx_hat output; dy_hat output
function [dx_hat,dy_hat] = EKF(timeTS,x,y,z,a_b,roll,pitch,yaw)

dt = 0.0025;


a_I = [(a_b(2)-sin(pitch))*cos(yaw)-sin(yaw)*((-a_b(1)-sin(roll)*cos(pitch)));
        sin(yaw)*(a_b(2)-sin(pitch))+cos(yaw)*((-a_b(1)-sin(roll)*cos(pitch)));
        a_b(3)-cos(roll)*cos(pitch)];

persistent time timeTS0 dx_k dP_k queue_dx queue_dP index Ndata timefreq
if isempty(dx_k) || isempty(dP_k)||isempty(time)|| isempty(timeTS0)|| isempty(queue_dx)|| isempty(queue_dP)|| isempty(index)|| isempty(timefreq)|| isempty(Ndata)

    dx_k = [0;0;0;0;z;0];  
    dP_k = eye(6,6);
    queue_dx = zeros(6,10);
    queue_dP = zeros(6,6,10);

    time = 0;
    timeTS0 = timeTS;
    index = 0;
    timefreq = 0;
    Ndata = 0;

else
    
    if timeTS~=0
        if timeTS0~=timeTS
            T = time;
            time = 0;
            timeTS0=timeTS;

            dF = [1 T  0 0  0 0;
                  0 1  0 0  0 0;
                  0 0  1 T  0 0;
                  0 0  0 1  0 0;
                  0 0  0 0  1 T;
                  0 0  0 0  0 1];
            dB = [0.5*T^2       0       0;
                       T        0       0;
                       0  0.5*T^2       0;
                       0        T       0;
                       0        0 0.5*T^2;
                       0        0       T];
            dw_k = [a_I(1);a_I(2);a_I(3)];
            dz_k = [x;y;z];
            dy_k = [dx_k(1);dx_k(3);dx_k(5)];
            dH =[1   0 0  0 0  0;
                0   0 1  0 0  0;
                0   0 0  0 1  0];
            dQ = diag([0 0.05  0 0.05 0 0.05]);
            dR = diag([0.001 0.001 0.001]);
            
        %---------PREDICTION---------%
        %1. Project the state ahead
            dx_k = dF * dx_k + dB * dw_k;
        %2. Project the error covariance ahead
            dP_k = dF * dP_k * dF' + dQ;  
        %--------CORRECTION----------%
        %1. Compute the Kalman Gain
            dK_k = dP_k * dH' / (dH*dP_k*dH' + dR);
            %resid = [sqrt(x0^2+y0^2);atan2(y0,x0);z0] - y_k;
            dresid = dz_k - dy_k;
        %2. Update the estimate via measurement
            dx_k = dx_k +dK_k * dresid;
        %3. Update the error covariance
            dP_k = (eye(size(dK_k,1)) - dK_k * dH) * dP_k;
            
            index = index + 1;

            if index > 10
                queue_dx(:,1) =  dx_k;
                queue_dP(:,:,1) = dP_k;
                index = 1;
            else
                queue_dx(:,index) =  dx_k;
                queue_dP(:,:,index) = dP_k;
            end

        else
            time = time + dt;
        end
   end  

end
dx_hat = dx_k(2);
dy_hat = dx_k(4);

== matlab function controlAerobi/Controllers/Quadrotor_Controllers/PID_cascade_controllers/PID_POSITION_CONTROLLER/XY_controller/create_references/Create dXY desired ==
  data: yaw input; chan2 input; chan3 input; dXY_d output
function dXY_d = dXYdesired(yaw,chan2,chan3)

R = [cos(yaw) -sin(yaw);sin(yaw) cos(yaw)];

dXY_d = R*[chan2;chan3];

== matlab function controlAerobi/Controllers/Quadrotor_Controllers/PID_cascade_controllers/PID_POSITION_CONTROLLER/XY_controller/Create RollPitchdesired ==
  data: yaw input; roll input; U input; ref output; r1 input; r2 input; p1 input; p2 input
function ref = RollPitchdesired(yaw,roll,U,r1,r2,p1,p2)

ref = [(1/9.81)*(r1*U(1)*sin(yaw) - r2*U(2)*cos(yaw));
       (1/(9.81*cos(roll)))*(p1*U(1)*cos(yaw)+p2*U(2)*sin(yaw))];
